simulink model "CarHalf_Verif"  (R2021b)
settings: Solver=VariableStepAuto  StartTime=0.0  StopTime=40  MaxStep=0.001  MinStep=0.0001  RelTol=1e-3
settings Model: Creator=Reece Bell  LastModifiedBy=reece
settings SolverCC: AlgebraicLoopSolver=TrustRegion
settings DataIOCC: ReturnWorkspaceOutputs=off
settings DebuggingCC: SFMachineParentedDataDiag=warning  ArithmeticOperatorsInVariantConditions=warning
settings SFSimCC: CustomCodeUndefinedFunction=UseInterfaceOnly

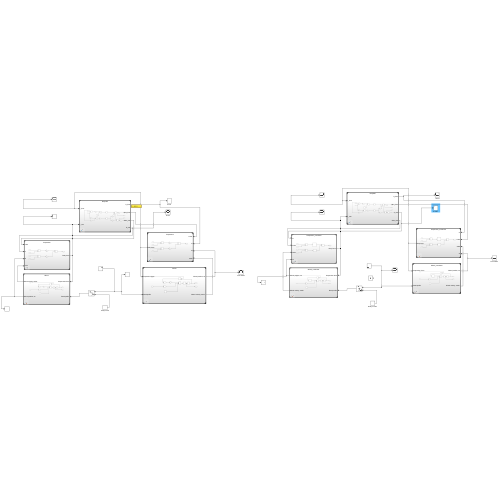
[thumbnail: Simulink's stored preview of the top-level diagram]
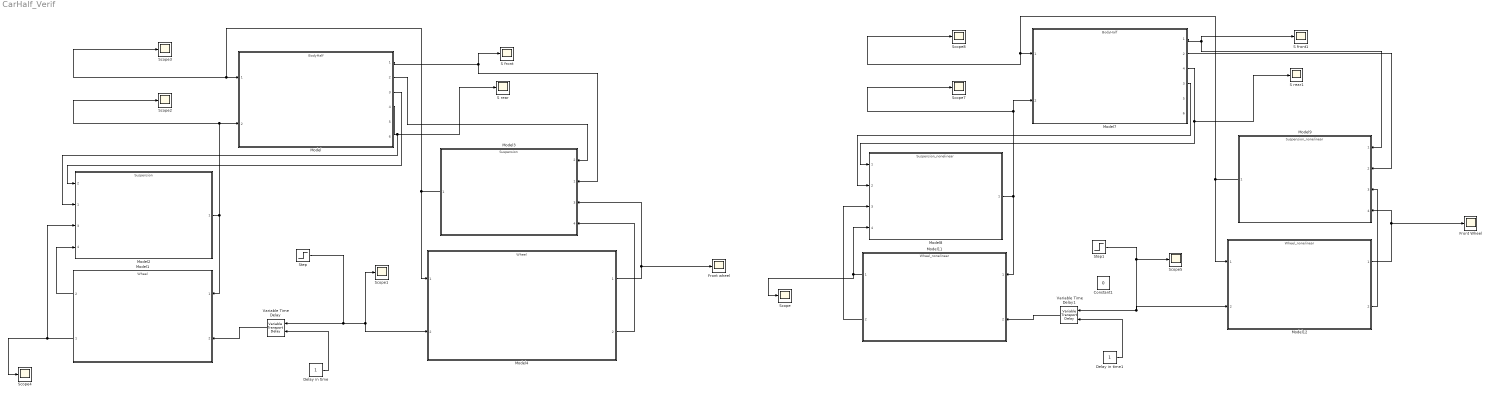
== system CarHalf_Verif ==
  Constant1 : Constant  Value=0
  Delay in time : Constant
  Delay in time1 : Constant
  Front Wheel : Scope
  Front wheel : Scope
  Model : ModelReference  ModelNameDialog=BodyHalf.slx  SimulationMode=Normal  ModelReferenceVersion=7.2
  Model1 : ModelReference  ModelNameDialog=Wheel.slx  SimulationMode=Normal  ModelReferenceVersion=1.11
      settings: PortSchema="{\"entries\":[{\"content\":{\"sides\":[{\"content\":{\"connectorIds\":[\"In1\",\"In2\"]},\"type\":\"ConnectorPlacement.EquallySpacedRectSide\",\"uuid\":\"71a4e87f-1851-4422-8936-4b87f85412fd\"},{\"content\":{\"connectorIds\":[\"Out2\",\"Out1\"],\"side\":\"RIGHT\"},\"type\":\"ConnectorPlacement.EquallySpacedRectSide\",\"uuid\":\"a8cbb71a-0d58-4894-b904-4ecd4e9fe1a2\"},{\"content\":{\"connectorIds\":[],\"side\":\"TOP\"},\"type\":\"ConnectorPlacement.EquallySpacedRectSide\",\"uuid\":\"1c77120d-7330-4516-954d-d61049980f4f\"}]},\"type\":\"ConnectorPlacement.EquallySpacedConnector\",\"uuid\":\"3f64bc7a-ba11-44ce-9e66-88e335d5dfb1\"}],\"packageUris\":[\"http://schema.mathworks.com/mf0/Connector/R2020b\"],\"version\":\"1.0\"}"
  Model11 : ModelReference  ModelNameDialog=Wheel_nonelinear.slx  SimulationMode=Normal  ModelReferenceVersion=1.17
  Model12 : ModelReference  ModelNameDialog=Wheel_nonelinear.slx  SimulationMode=Normal  ModelReferenceVersion=1.17
  Model2 : ModelReference  ModelNameDialog=Suspension.slx  SimulationMode=Normal  ModelReferenceVersion=1.8
      settings: PortSchema="{\"entries\":[{\"content\":{\"sides\":[{\"content\":{\"connectorIds\":[\"In2\",\"In1\",\"In3\",\"In4\"]},\"type\":\"ConnectorPlacement.EquallySpacedRectSide\",\"uuid\":\"94601151-747d-4428-9167-f5fe05b2d5ec\"},{\"content\":{\"connectorIds\":[\"Out1\"],\"side\":\"RIGHT\"},\"type\":\"ConnectorPlacement.EquallySpacedRectSide\",\"uuid\":\"dff19792-31ea-4015-87a5-b27b5b8418bd\"},{\"content\":{\"connectorIds\":[],\"side\":\"TOP\"},\"type\":\"ConnectorPlacement.EquallySpacedRectSide\",\"uuid\":\"ecb08bd5-caa0-4733-8680-fe03693d318b\"}]},\"type\":\"ConnectorPlacement.EquallySpacedConnector\",\"uuid\":\"5a835372-3a50-49f7-b808-dc60be46a96a\"}],\"packageUris\":[\"http://schema.mathworks.com/mf0/Connector/R2020b\"],\"version\":\"1.0\"}"
  Model3 : ModelReference  ModelNameDialog=Suspension.slx  SimulationMode=Normal  ModelReferenceVersion=1.8
      settings: PortSchema="{\"entries\":[{\"content\":{\"sides\":[{\"content\":{\"connectorIds\":[\"In2\",\"In1\",\"In3\",\"In4\"]},\"type\":\"ConnectorPlacement.EquallySpacedRectSide\",\"uuid\":\"94601151-747d-4428-9167-f5fe05b2d5ec\"},{\"content\":{\"connectorIds\":[\"Out1\"],\"side\":\"RIGHT\"},\"type\":\"ConnectorPlacement.EquallySpacedRectSide\",\"uuid\":\"dff19792-31ea-4015-87a5-b27b5b8418bd\"},{\"content\":{\"connectorIds\":[],\"side\":\"TOP\"},\"type\":\"ConnectorPlacement.EquallySpacedRectSide\",\"uuid\":\"ecb08bd5-caa0-4733-8680-fe03693d318b\"}]},\"type\":\"ConnectorPlacement.EquallySpacedConnector\",\"uuid\":\"5a835372-3a50-49f7-b808-dc60be46a96a\"}],\"packageUris\":[\"http://schema.mathworks.com/mf0/Connector/R2020b\"],\"version\":\"1.0\"}"
  Model4 : ModelReference  ModelNameDialog=Wheel.slx  SimulationMode=Normal  ModelReferenceVersion=1.11
  Model7 : ModelReference  ModelNameDialog=BodyHalf.slx  SimulationMode=Normal  ModelReferenceVersion=7.2
      settings: PortSchema="{\"entries\":[{\"content\":{\"sides\":[{\"content\":{\"connectorIds\":[\"In1\",\"In2\"]},\"type\":\"ConnectorPlacement.EquallySpacedRectSide\",\"uuid\":\"170361de-c344-42bb-ab42-af554e1f149d\"},{\"content\":{\"connectorIds\":[\"Out1\",\"Out2\",\"Out4\",\"Out3\",\"Out5\",\"Out6\"],\"side\":\"RIGHT\"},\"type\":\"ConnectorPlacement.EquallySpacedRectSide\",\"uuid\":\"321b32d6-c6a2-4ac8-b82c-5f88b7662cfd\"},{\"content\":{\"connectorIds\":[],\"side\":\"TOP\"},\"type\":\"ConnectorPlacement.EquallySpacedRectSide\",\"uuid\":\"5f859d15-1c1e-4242-9cc2-f1cb99b438b7\"}]},\"type\":\"ConnectorPlacement.EquallySpacedConnector\",\"uuid\":\"eb5cce4d-7e0f-42cd-b6e0-3c17456a4040\"}],\"packageUris\":[\"http://schema.mathworks.com/mf0/Connector/R2020b\"],\"version\":\"1.0\"}"
  Model8 : ModelReference  ModelNameDialog=Suspension_nonelinear.slx  SimulationMode=Normal  ModelReferenceVersion=1.12
  Model9 : ModelReference  ModelNameDialog=Suspension_nonelinear.slx  SimulationMode=Normal  ModelReferenceVersion=1.12
  S front : Scope
  S front1 : Scope
  S rear : Scope
  S rear1 : Scope
  Scope{,1..5,7..8} (8 alike) : Scope
  Step : Step  SampleTime=0
  Step1 : Step  SampleTime=0
  Variable Time Delay : VariableTransportDelay  MaximumDelay=10  ZeroDelay=on
  Variable Time Delay1 : VariableTransportDelay  MaximumDelay=10  ZeroDelay=on
  wires:
  Step/1 -> Variable Time Delay/1, Scope1/1, Model4/2
  Delay in time/1 -> Variable Time Delay/2
  Model2/1 -> Model1/1, Model/2, Scope2/1
  Model3/1 -> Model4/1, Scope3/1, Model/1
  Variable Time Delay/1 -> Model1/2
  Model4/2 -> Model3/4
  Model/1 -> Model3/1, S front/1
  Model/2 -> Model3/2
  Variable Time Delay1/1 -> Model11/2
  Model8/1 -> Model7/2, Scope7/1, Model11/1
  Model9/1 -> Model12/1, Scope8/1, Model7/1
  Delay in time1/1 -> Variable Time Delay1/2
  Model4/1 -> Front wheel/1, Model3/3
  Model1/1 -> Scope4/1, Model2/3
  Model1/2 -> Model2/4
  Model/3 -> Model2/2
  Model/4 -> S rear/1, Model2/1
  Model7/1 -> Model9/1, S front1/1
  Model7/4 -> Model8/1, S rear1/1
  Model7/2 -> Model9/2
  Model12/1 -> Front Wheel/1, Model9/4
  Model12/2 -> Model9/3
  Model11/1 -> Model8/4, Scope/1
  Model11/2 -> Model8/3
  Model7/3 -> Model8/2
  Step1/1 -> Scope5/1, Model12/2, Variable Time Delay1/1
